simulink model "hardware3"  (R2018a)
settings: Solver=VariableStepDiscrete  StartTime=0.0  StopTime=5  RelTol=1e-3  EnableMultiTasking=on
libraries: powerlib x11
settings Model: Creator=Hakan Polat  LastModifiedBy=Onur
settings OptimizationCC: LifeSpan=inf
settings DebuggingCC: MaxConsecutiveZCsMsg=none  SFUnexpectedBacktrackingDiag=warning  SFNoUnconditionalDefaultTransitionDiag=warning  SFExecutionAtInitializationDiag=none
settings CodeAppCC: StateflowObjectComments=on
settings GRTTargetCC: TargetLangStandard=C89/C90 (ANSI)  GeneratePreprocessorConditionals=Disable all
settings ConfigComp: CovMetricSettings=dw  CovHtmlReporting=on  CovSaveCumulativeToWorkspaceVar=on  CovSaveSingleToWorkspaceVar=on  CovExternalEMLEnable=off
settings SimscapeCC: SimscapeNormalizeSystem=off

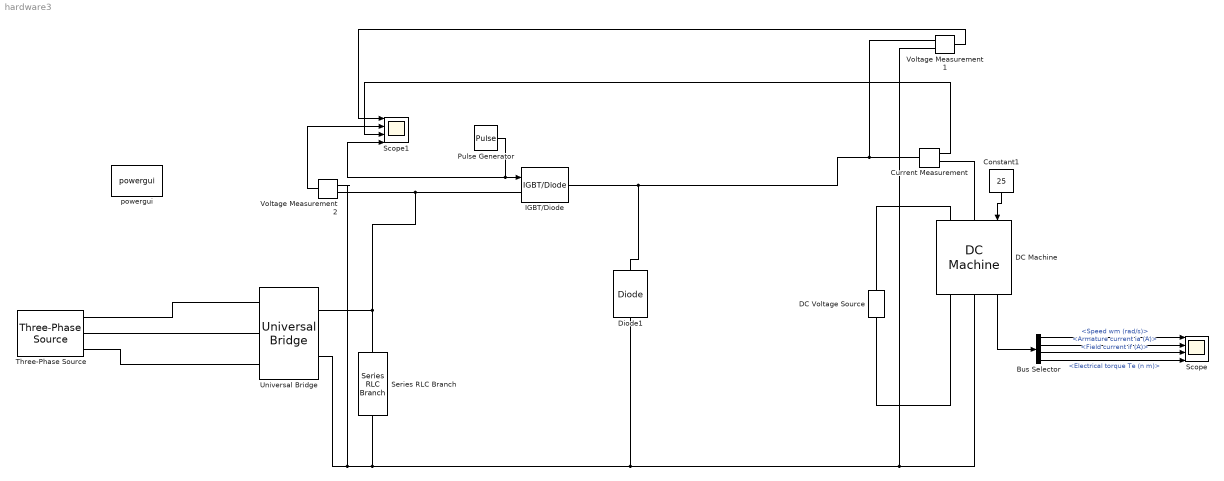
== system hardware3 ==
  Bus Selector : BusSelector  OutputSignals=Speed wm (rad/s),Armature current ia (A),Field current if (A),Electrical torque Te (n m)
  Constant1 : Constant  Value=25
  Current Measurement : powerlib/Measurements/Current Measurement  PhasorSimulation=off  OutputType=Complex  PSBequivalent=0
  DC Machine : powerlib/Machines/DC Machine  PresetModel=No  MechanicalLoad=Torque TL  FieldType=Wound  ShowDetailedParameters=on  MeasurementBus=off  RLa="[ 0.8  0.0125]"  RLf="[ 210  23]"  Laf=1.8  MachineConstant=Torque constant (N.m/A)  Ke=1.8  Kt=1.8  J=1  Bm=0  Tf=0  w0=0  Ifinit=1  TsPowergui=0  TsBlock=-1
  DC Voltage Source : powerlib/Electrical Sources/DC Voltage Source  Amplitude=150  Measurements=None
  Diode1 : powerlib/Power Electronics/Diode  Ron=0.001  Lon=0  Vf=0.8  IC=0  UseSnubber=off  Rs=500  Cs=250e-9  Measurements=off
  IGBT/Diode : powerlib/Power Electronics/IGBT//Diode  Ron=1e-3  Rs=27  Cs=9e-9  Measurements=off
  Pulse Generator : DiscretePulseGenerator  PulseType=Time based  Amplitude=10  Period=1/3900  PulseWidth=30
  Scope : Scope  NumInputPorts=4
  Scope1 : Scope  NumInputPorts=4
  Series RLC Branch : powerlib/Elements/Series RLC Branch  LConnTagsString=__new0  RConnTagsString=__new0  BranchType=C  Resistance=1  Inductance=1e-3  SetiL0=off  InitialCurrent=0  Capacitance=940e-6  Setx0=off  InitialVoltage=0  Measurements=None
  Three-Phase Source : powerlib/Electrical Sources/Three-Phase Source  InternalConnection=Yg  VoltagePhases=off  Voltage=150  PhaseAngle=0  Voltage_phases=[25e3 25e3 25e3]/sqrt(3)  PhaseAngles_phases=[0 -120 +120]  Frequency=50  NonIdealSource=on  SpecifyImpedance=off  Resistance=100e-3  Inductance=100e-6  ShortCircuitLevel=100e6  BaseVoltage=0  XRratio=7  BusType=swing  Pref=10e3  Qref=0  Prefabc=[10e3, 10e3, 10e3]  Qrefabc=[0, 0, 0]  Qmin=-inf  Qmax=inf
  Universal Bridge : powerlib/Power Electronics/Universal Bridge  Arms=3  SnubberResistance=1e5  SnubberCapacitance=inf  Device=Diodes  Ron=20e-3  Lon=0  ForwardVoltages="[  0  0  ]"  ForwardVoltage=0.8  GTOparameters=[ 10e-6 , 20e-6 ]  IGBTparameters=[ 1e-6 , 2e-6 ]  Measurements=None  Measurements_2=None  converterType=Rectifier
  Voltage Measurement1 : powerlib/Measurements/Voltage Measurement  PhasorSimulation=off  OutputType=Complex  PSBequivalent=0
  Voltage Measurement2 : powerlib/Measurements/Voltage Measurement  PhasorSimulation=off  OutputType=Complex  PSBequivalent=0
  powergui : powerlib/powergui  Priority=1  SimulationMode=Discrete  SampleTime=1e-6  frequency=60  Iterations=50  frequencyindice=0  Pbase=100e6  ErrMax=1e-4  UnitsV=kV  UnitsW=MW  buscounter=0  FunctionMessages=off  echomessages=off  EnableUseOfTLC=off  CurrentSourceSwitches=off  DisableSnubberDevices=off  DisableRonSwitches=off  DisableVfSwitches=off  DisplayEquations=off  SolverType=Tustin/Backward Euler (TBE)  Interpol=off  ExternalGateDelay=off  methode=off  Ts=100  x0status=blocks  SPID=off  SwTol=0  HookPort=off  RestoreLinks=warning  ResistiveCurrentMeasurement=off  Frange=[0:2:500]  Ylog=off  Xlog=on  ShowGrid=off  save=off  variable=ZData  structure=0  ZoomFFT=off  StartTime=0.0  cycles=1  DisplayStyle=1  fundamental=60  FreqAxis=off  MaxFrequency=1000  frequencyindicesteady=1  RmsSteady=1  display=off
  wires:
  Constant1/1 -> DC Machine/1
  DC Machine/1 -> Bus Selector/1
  Bus Selector/1 -> Scope/1  "<Speed wm (rad/s)>"
  Bus Selector/2 -> Scope/2  "<Armature current ia (A)>"
  Bus Selector/3 -> Scope/3  "<Field current if (A)>"
  Bus Selector/4 -> Scope/4  "<Electrical torque Te (n m)>"
  Voltage Measurement2/1 -> Scope1/2
  Current Measurement/1 -> Scope1/3
  Pulse Generator/1 -> Scope1/4, IGBT/Diode/1
  Voltage Measurement1/1 -> Scope1/1
  connections:
  Universal Bridge/LConn2 -- Three-Phase Source/RConn2
  Universal Bridge/LConn3 -- Three-Phase Source/RConn3
  Universal Bridge/RConn2 -- Voltage Measurement1/LConn2 -- DC Machine/RConn1 -- Diode1/LConn1 -- Series RLC Branch/RConn1 -- Voltage Measurement2/LConn2
  Three-Phase Source/RConn1 -- Universal Bridge/LConn1
  Universal Bridge/RConn1 -- IGBT/Diode/LConn1 -- Voltage Measurement2/LConn1 -- Series RLC Branch/LConn1
  DC Voltage Source/LConn1 -- DC Machine/RConn2
  DC Machine/LConn2 -- DC Voltage Source/RConn1
  DC Machine/LConn1 -- Current Measurement/RConn1
  IGBT/Diode/RConn1 -- Diode1/RConn1 -- Voltage Measurement1/LConn1 -- Current Measurement/LConn1
